simulink model "RGB2gray"  (R2023b)
settings: Solver=VariableStepAuto  StartTime=0.0  StopTime=10.0  RelTol=1e-3
libraries: visionsources x1
settings Model: Creator=trzp  LastModifiedBy=trzp

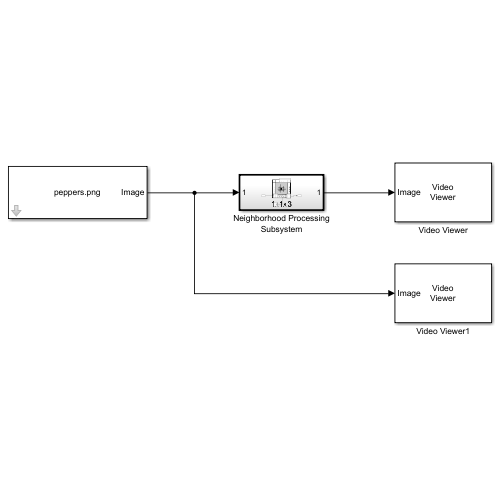
[thumbnail: Simulink's stored preview of the top-level diagram]
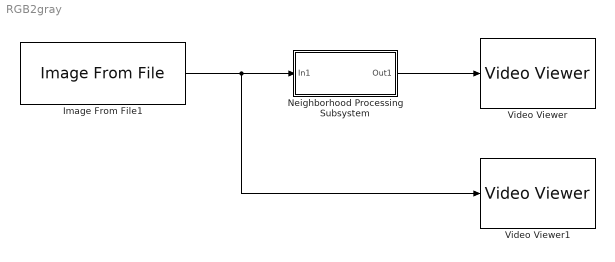
== system RGB2gray ==
  Image From File1 : visionsources/Image From File  Tag=vipblks_nd  FileName=peppers.png  Ts=inf  imagePorts=One multidimensional signal  OutPortLabels=R|G|B  ImageDataType=double  sdImageDataType=uint(8)  Signed=on  WordLength=16  FractionLengthMode=User-defined  FractionLength=15
  Neighborhood Processing Subsystem : Subsystem  TreatAsAtomicUnit=on
  Video Viewer : VideoViewer  FigPos=[675.4 790 417.6 304]
  Video Viewer1 : VideoViewer  FigPos=[245 540.4 417.6 304]
  wires:
  Neighborhood Processing Subsystem/1(Out1) -> Video Viewer/1
  Image From File1/1 -> Video Viewer1/1, Neighborhood Processing Subsystem/1(In1)

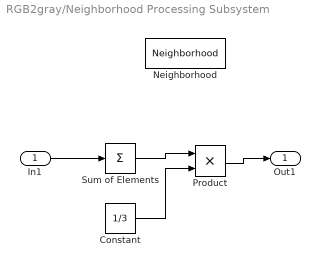
== system RGB2gray/Neighborhood Processing Subsystem ==
  In1 : Inport
  Constant : Constant  Value=1/3
  Neighborhood : Neighborhood  NeighborhoodSize=[1 1 3]  Stride=[1 1 1]  ProcessingOffset=[0 0 0]  OutputSize=Valid
  Product : Product
  Sum of Elements : Sum  Inputs=+
  Out1 : Outport  ConcatenationDimension=[1 2]
  wires:
  In1/1 -> Sum of Elements/1
  Product/1 -> Out1/1
  Sum of Elements/1 -> Product/1
  Constant/1 -> Product/2
